simulink library "RASPlib"  (R2015a)
settings: Solver=ode45  StartTime=0.0  StopTime=10.0  RelTol=1e-3
PostLoadFcn:
  | setsysloc(bdroot)
StartFcn:
  | open_system('MinSegLibrary','force')
libraries: arduinolib x3
settings Model: Creator=hurstj  LastModifiedBy=Administrator
settings DataIOCC: SignalLoggingSaveFormat=ModelDataLogs
settings DebuggingCC: UnderspecifiedInitializationDetection=Classic  MergeDetectMultiDrivingBlocksExec=none  SolverPrmCheckMsg=warning  MultiTaskDSMMsg=warning  MultiTaskCondExecSysMsg=none  StateNameClashWarn=warning  StrictBusMsg=None

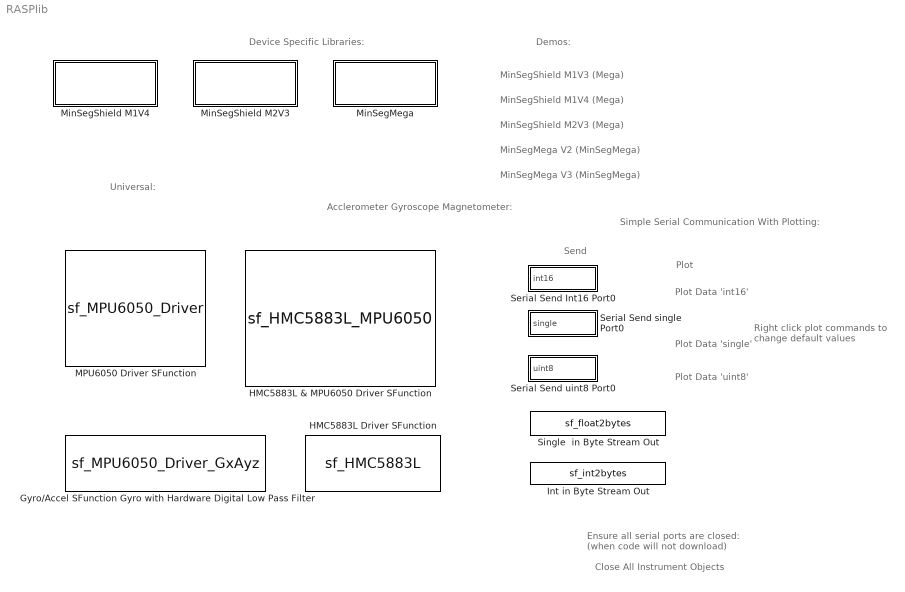
== system RASPlib ==
  note: Right click
      |  plot commands
      | to change
      | default values
  note: Ensure all serial ports are closed:
      | (when code will not download)
  note: Plot
  note: Send
  note: Device Specific Libraries:
  note: MinSegShield M1V3 (Mega)
  note: Plot Data
      | 'int16'
  note: Plot Data
      | 'single'
  note: Plot Data
      | 'uint8'
  note: MinSegShield M1V4 (Mega)
  note: MinSegShield M2V3 (Mega)
  note: MinSegMega V2 (MinSegMega)
  note: MinSegMega V3 (MinSegMega)
  note: Universal:
  note: Acclerometer Gyroscope
      | Magnetometer:
  note: Simple Serial Communication
      | With Plotting:
  note: Demos:
  note: Close All
      | Instrument Objects
  Gyro/Accel SFunction Gyro with Hardware Digital Low Pass Filter : S-Function  InitFcn=try, set_param(gcb,'FunctionName','sf_MPU6050_Driver_GxAyz'), end  FunctionName=sf_MPU6050_Driver_GxAyz  SFunctionModules=sf_MPU6050_Driver_GxAyz_wrapper  mask(S-Function Builder){}
      mask help: Simulink:masks:SFunctionBuilder_MD
      mask init:
      | val = [[.9  0.75 0.75 1 1 .9 .9 1]',[1 1 0.75 0.75 .9 .9 1 .9]'];try , sys = get_param(gcb,'SfunBuilderFcnName');if isempty(sys), sys = get_param(gcb,'FunctionName'); end,catch, sys = get_param(gcb,'FunctionName'); end
      settings: CopyFcn=set_param(gcbh,'LinkStatus','none')  PreSaveFcn=try, set_param(gcb,'FunctionName','sf_MPU6050_Driver_GxAyz'), end  OpenFcn=sfunctionwizard(gcbh)
      mask Display: plot(val(:,1),val(:,2)),disp(sys), port_label('output',1,'x_vel'), port_label('output',2,'y_acc'), port_label('output',3,'z_acc')
  HMC5883L & MPU6050 Driver SFunction : S-Function  InitFcn=try, set_param(gcb,'FunctionName','sf_HMC5883L_MPU6050'), end  FunctionName=sf_HMC5883L_MPU6050  SFunctionModules=sf_HMC5883L_MPU6050_wrapper  mask(S-Function Builder){}
      mask help: Simulink:masks:SFunctionBuilder_MD
      mask init: same as RASPlib/Gyro/Accel SFunction Gyro with Hardware Digital Low Pass Filter
      settings: CopyFcn=set_param(gcbh,'LinkStatus','none')  PreSaveFcn=try, set_param(gcb,'FunctionName','sf_HMC5883L_MPU6050'), end  OpenFcn=sfunctionwizard(gcbh)
      mask Display: plot(val(:,1),val(:,2)),disp(sys), port_label('output',1,'x_mag'), port_label('output',2,'y_mag'), port_label('output',3,'z_mag'), port_label('output',4,'x_vel'), port_label('output',5,'y_vel'), port_label('output',6,'z_vel'), port_label('output',7,'x_acc'), port_label('output',8,'y_acc'), port_label('output',9,'z_acc')
  HMC5883L Driver SFunction : S-Function  InitFcn=try, set_param(gcb,'FunctionName','sf_HMC5883L'), end  FunctionName=sf_HMC5883L  SFunctionModules=sf_HMC5883L_wrapper  mask(S-Function Builder){}
      mask help: Simulink:masks:SFunctionBuilder_MD
      mask init: same as RASPlib/Gyro/Accel SFunction Gyro with Hardware Digital Low Pass Filter
      settings: CopyFcn=set_param(gcbh,'LinkStatus','none')  PreSaveFcn=try, set_param(gcb,'FunctionName','sf_HMC5883L'), end  OpenFcn=sfunctionwizard(gcbh)
      mask Display:
      | plot(val(:,1),val(:,2))
      | disp(sys)
      | port_label('output',1,'x_val')
      | port_label('output',2,'y_val')
      | port_label('output',3,'z_val')
  Int in Byte Stream Out : S-Function  InitFcn=try, set_param(gcb,'FunctionName','sf_int2bytes'), end  FunctionName=sf_int2bytes  SFunctionModules=sf_int2bytes_wrapper  mask(S-Function Builder){}
      mask init: same as RASPlib/Gyro/Accel SFunction Gyro with Hardware Digital Low Pass Filter
      settings: CopyFcn=set_param(gcb,'LinkStatus','none')  PreSaveFcn=try, set_param(gcb,'FunctionName','sf_int2bytes'), end  OpenFcn=sfunctionwizard(gcbh)
      mask Display: plot(val(:,1),val(:,2)),disp(sys), port_label('input',1,'int_in'), port_label('output',1,'bout')
  MPU6050 Driver SFunction : S-Function  InitFcn=try, set_param(gcb,'FunctionName','sf_MPU6050_Driver'), end  FunctionName=sf_MPU6050_Driver  SFunctionModules=sf_MPU6050_Driver_wrapper  mask(S-Function Builder){}
      mask help: Simulink:masks:SFunctionBuilder_MD
      mask init: same as RASPlib/Gyro/Accel SFunction Gyro with Hardware Digital Low Pass Filter
      settings: CopyFcn=set_param(gcbh,'LinkStatus','none')  PreSaveFcn=try, set_param(gcb,'FunctionName','sf_MPU6050_Driver'), end  OpenFcn=sfunctionwizard(gcbh)
      mask Display: plot(val(:,1),val(:,2)),disp(sys), port_label('output',1,'x_vel'), port_label('output',2,'y_vel'), port_label('output',3,'z_vel'), port_label('output',4,'x_acc'), port_label('output',5,'y_acc'), port_label('output',6,'z_acc')
  MinSegMega : Subsystem
      settings: OpenFcn=MinSegLibrary_MinSegMega
      mask Display: disp('MinSegMega')
  MinSegShield M1V4 : Subsystem
      settings: OpenFcn=MinSegLibrary_M1V4
      mask Display: disp('MinSegShield\nM1V4')
  MinSegShield M2V3 : Subsystem
      settings: OpenFcn=MinSegLibrary_M2V3
      mask Display: disp('MinSegShield\nM2V3')
  Serial Send Int16 Port0 : Subsystem
  Serial Send single Port0 : Subsystem
  Serial Send uint8 Port0 : Subsystem
  Single  in Byte Stream Out : S-Function  InitFcn=try, set_param(gcb,'FunctionName','sf_float2bytes'), end  FunctionName=sf_float2bytes  SFunctionModules=sf_float2bytes_wrapper  mask(S-Function Builder){}
      mask init: same as RASPlib/Gyro/Accel SFunction Gyro with Hardware Digital Low Pass Filter
      settings: CopyFcn=set_param(gcb,'LinkStatus','none')  PreSaveFcn=try, set_param(gcb,'FunctionName','sf_float2bytes'), end  OpenFcn=sfunctionwizard(gcbh)
      mask Display: plot(val(:,1),val(:,2)),disp(sys), port_label('input',1,'fin'), port_label('output',1,'bout')

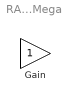
== system RASPlib/MinSegMega ==
  Gain : Gain

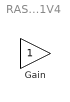
== system RASPlib/MinSegShield M1V4 ==
  Gain : Gain

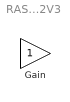
== system RASPlib/MinSegShield M2V3 ==
  Gain : Gain

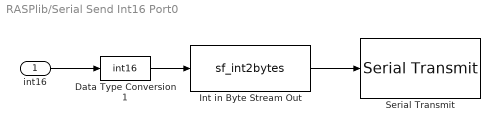
== system RASPlib/Serial Send Int16 Port0 ==
  int16 : Inport
  Data Type Conversion1 : DataTypeConversion  OutDataTypeStr=int16
  Int in Byte Stream Out : S-Function  InitFcn=try, set_param(gcb,'FunctionName','sf_int2bytes'), end  FunctionName=sf_int2bytes  SFunctionModules=sf_int2bytes_wrapper  mask(S-Function Builder){}
      mask init: same as RASPlib/Gyro/Accel SFunction Gyro with Hardware Digital Low Pass Filter
      settings: CopyFcn=set_param(gcb,'LinkStatus','none')  PreSaveFcn=try, set_param(gcb,'FunctionName','sf_int2bytes'), end  OpenFcn=sfunctionwizard(gcbh)
      mask Display: plot(val(:,1),val(:,2)),disp(sys), port_label('input',1,'int_in'), port_label('output',1,'bout')
  Serial Transmit : arduinolib/Serial Transmit  portNumber=0
  wires:
  Data Type Conversion1/1 -> Int in Byte Stream Out/1
  int16/1 -> Data Type Conversion1/1
  Int in Byte Stream Out/1 -> Serial Transmit/1

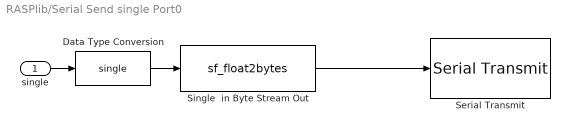
== system RASPlib/Serial Send single Port0 ==
  single : Inport
  Data Type Conversion : DataTypeConversion  OutDataTypeStr=single
  Serial Transmit : arduinolib/Serial Transmit  portNumber=0
  Single  in Byte Stream Out : S-Function  InitFcn=try, set_param(gcb,'FunctionName','sf_float2bytes'), end  FunctionName=sf_float2bytes  SFunctionModules=sf_float2bytes_wrapper  mask(S-Function Builder){}
      mask init: same as RASPlib/Gyro/Accel SFunction Gyro with Hardware Digital Low Pass Filter
      settings: CopyFcn=set_param(gcb,'LinkStatus','none')  PreSaveFcn=try, set_param(gcb,'FunctionName','sf_float2bytes'), end  OpenFcn=sfunctionwizard(gcbh)
      mask Display: plot(val(:,1),val(:,2)),disp(sys), port_label('input',1,'fin'), port_label('output',1,'bout')
  wires:
  Data Type Conversion/1 -> Single  in Byte Stream Out/1
  single/1 -> Data Type Conversion/1
  Single  in Byte Stream Out/1 -> Serial Transmit/1

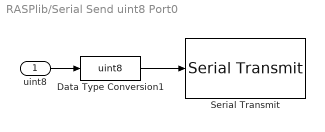
== system RASPlib/Serial Send uint8 Port0 ==
  uint8 : Inport
  Data Type Conversion1 : DataTypeConversion  OutDataTypeStr=uint8
  Serial Transmit : arduinolib/Serial Transmit  portNumber=0
  wires:
  uint8/1 -> Data Type Conversion1/1
  Data Type Conversion1/1 -> Serial Transmit/1
